simulink subsystem "SOH_single_cell"  (R2024a)
settings: Solver=VariableStepAuto  StartTime=0.0  StopTime=10.0  RelTol=1e-3
values from neighbouring files (symbols this model uses):
  cap_measurement_covariance = 5.0E-7    [EstimatorsDictionary.sldd]
  cell_capacity_nominal = 116.0    [CellDictionary.sldd]    (also in Gotion116CellDictionary.sldd)
  Ts = 1.0    [EstimatorsDictionary.sldd]    (also in batteryStateTransition.m = u(3))
libraries: BatteryEstimators x5
settings Model: DataDictionary=EstimatorsDictionary.sldd  EnableAccessToBaseWorkspace=off  Creator=mmackenzie  LastModifiedBy=mmackenzie

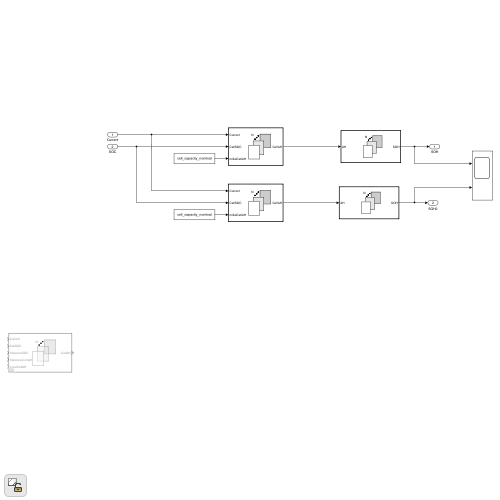
[thumbnail: Simulink's stored preview of the top-level diagram]
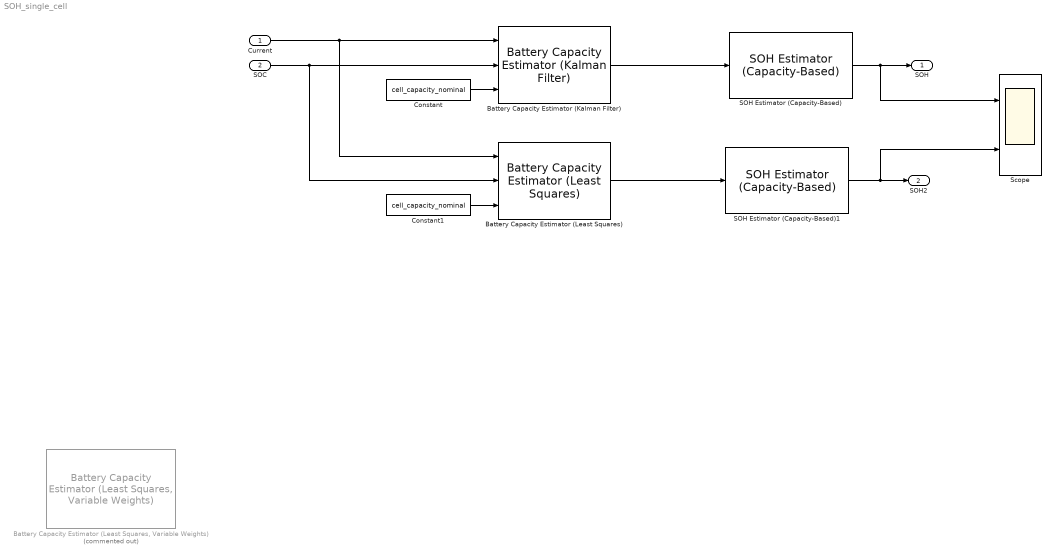
== system SOH_single_cell ==
  Current : Inport
  SOC : Inport  Port=2
  Battery Capacity Estimator (Kalman Filter) : BatteryEstimators/Battery Capacity Estimator (Kalman Filter)  CurrentInputPartition=off  filterType=Extended Kalman filter  alpha=1  beta=2  kappa=0  Q=cap_process_covariance  R=cap_measurement_covariance  P0=cap_initial_covariance  Ts=Ts
      settings: LibrarySourceBlock=|
      | batt_sl_lib/Estimators/Battery Capacity Estimator
      | (Kalman Filter)
  Battery Capacity Estimator (Least Squares) : BatteryEstimators/Battery Capacity Estimator (Least Squares)  CurrentInputPartition=off  lsAlgorithm=Ordinary least squares  SocChangeThreshold=cap_soc_change_threshold  gamma=cap_forgetting_factor  VarianceX=2e-4  VarianceY=cap_current_measurement_variance  k=10  Ts=Ts
      settings: LibrarySourceBlock=|
      | batt_sl_lib/Estimators/Battery Capacity Estimator
      | (Least Squares)
  "Battery Capacity Estimator (Least Squares, Variable Weights)" : BatteryEstimators/Battery Capacity Estimator (Least Squares, Variable Weights)  Commented=on  CurrentInputPartition=off  lsAlgorithm=Ordinary least squares  SocChangeThreshold=0.03  gamma=0.9  k=20  Ts=1
      settings: LibrarySourceBlock=|
      | batt_sl_lib/Estimators/Battery Capacity Estimator
      | (Least Squares, Variable Weights)
  Constant : Constant  Value=cell_capacity_nominal
  Constant1 : Constant  Value=cell_capacity_nominal
  SOH Estimator (Capacity-Based) : BatteryEstimators/SOH Estimator (Capacity-Based)  AH_new=cell_capacity_nominal  AH_eol=1e-6
      settings: LibrarySourceBlock=batt_sl_lib/Estimators/SOH Estimator (Capacity-Based)
  SOH Estimator (Capacity-Based)1 : BatteryEstimators/SOH Estimator (Capacity-Based)  AH_new=cell_capacity_nominal  AH_eol=1e-6
      settings: LibrarySourceBlock=batt_sl_lib/Estimators/SOH Estimator (Capacity-Based)
  Scope : Scope  NumInputPorts=2
  SOH : Outport
  SOH2 : Outport  Port=2
  wires:
  SOH Estimator (Capacity-Based)/1 -> Scope/1, SOH/1
  Battery Capacity Estimator (Kalman Filter)/1 -> SOH Estimator (Capacity-Based)/1
  Battery Capacity Estimator (Least Squares)/1 -> SOH Estimator (Capacity-Based)1/1
  SOH Estimator (Capacity-Based)1/1 -> SOH2/1, Scope/2
  Current/1 -> Battery Capacity Estimator (Least Squares)/1, Battery Capacity Estimator (Kalman Filter)/1
  SOC/1 -> Battery Capacity Estimator (Least Squares)/2, Battery Capacity Estimator (Kalman Filter)/2
  Constant/1 -> Battery Capacity Estimator (Kalman Filter)/3
  Constant1/1 -> Battery Capacity Estimator (Least Squares)/3
